simulink model "PID_Controller"  (R2020a)
settings: Solver=VariableStepAuto  StartTime=0.0  StopTime=120  RelTol=1e-3
settings Model: DataDictionary=Week2_Problem3.sldd  Creator=sreeram  LastModifiedBy=sreeram
settings DataIOCC: SaveOutput=off  SaveTime=off

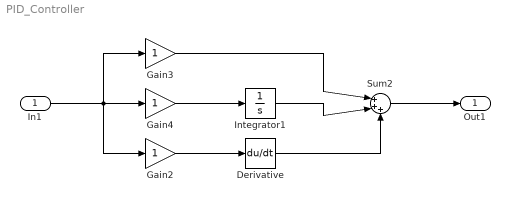
== system PID_Controller ==
  In1 : Inport  OutDataTypeStr=double  PortDimensions=1  SampleTime=0
  Derivative : Derivative
  Gain2 : Gain
  Gain3 : Gain
  Gain4 : Gain
  Integrator1 : Integrator
  Sum2 : Sum  Inputs=|+++
  Out1 : Outport  OutDataTypeStr=double  PortDimensions=1  SampleTime=0
  wires:
  Gain3/1 -> Sum2/1
  In1/1 -> Gain4/1, Gain3/1, Gain2/1
  Sum2/1 -> Out1/1
  Gain4/1 -> Integrator1/1
  Derivative/1 -> Sum2/3
  Integrator1/1 -> Sum2/2
  Gain2/1 -> Derivative/1
